simulink model "A3_control_loop_lin_d_model"  (Simulink 8.7)
settings: Solver=VariableStepDiscrete  StartTime=0.0  StopTime=5  MaxStep=1e-3  RelTol=1e-3
values from neighbouring files (symbols this model uses):
  H = sum_H * lin_sys.b    [a2_main.m]    (also in a3_main.m; a4_main.m)
  K_I = 0.31    [a3_main.m]    (also in a4_main.m)
  K_M = 1/63000    (= 1.5873015873e-05)    [a1_main.m]    (also in a2_main.m; a3_main.m; a4_main.m)
  lin_sys = linmod('A1_Hydropulszylinder',zeros(3,1),0)    [a1_main.m]    (also in a2_main.m; a3_main.m; a4_main.m)
  PHI = expm(Ta*lin_sys.a)    [a2_main.m]    (also in a3_main.m; a4_main.m)
  Ta = 15e-3    (= 0.015)    [a1_main.m]    (also in a2_main.m; a3_main.m; a4_main.m)
undefined symbols (not defined in the file or in its folder): DiscIntNeverNeededParam
libraries: simulink x1
settings Model: Creator=jinyao  LastModifiedBy=jinyao
settings DataIOCC: LimitDataPoints=off  SaveFormat=Dataset
settings DebuggingCC: UnderspecifiedInitializationDetection=Simplified  MergeDetectMultiDrivingBlocksExec=error
settings HardwareCC: ProdBitPerPointer=64  ProdLargestAtomicFloat=Float  ProdIntDivRoundTo=Zero  ProdEndianess=LittleEndian  ProdWordSize=64  ProdHWDeviceType=Intel->x86-64 (Windows64)
settings ModelReferenceCC: PropagateSignalLabelsOutOfModel=on
settings ConfigComp: CovModelRefEnable=off

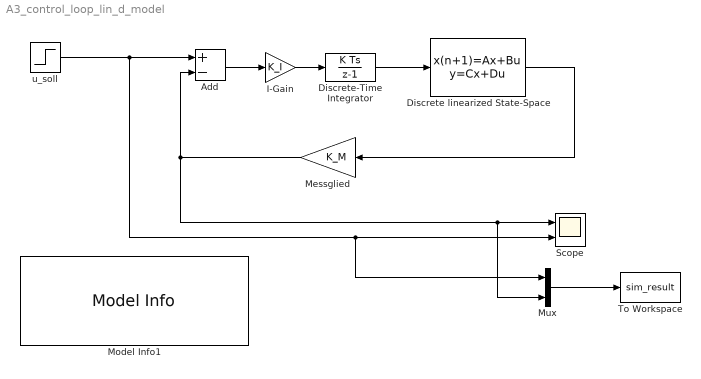
== system A3_control_loop_lin_d_model ==
  Add : Sum  Inputs=+-
  Discrete linearized State-Space : DiscreteStateSpace  A=PHI  B=H  C=lin_sys.c  D=0  SampleTime=Ta
  Discrete-Time Integrator : DiscreteIntegrator  InitialConditionSetting=State (most efficient)  SampleTime=Ta  ICPrevOutput=DiscIntNeverNeededParam  ICPrevScaledInput=DiscIntNeverNeededParam
  I-Gain : Gain  Gain=K_I
  Messglied : Gain  Gain=K_M
  Model Info1 : simulink/Model-Wide Utilities/Model Info  Frame=on  DisplayStringWithTags=|  HorizontalTextAlignment=Center  LeftAlignmentValue=0.5  SourceBlockDiagram=A3_control_loop_lin_d_model  TagMaxNumber=20
      | %<ModelName>
      | 
      | MODSIM GRUPPE 11
      | 
      | Cao,Bozhi  Gao,Yue  Jia,Xuehua  Zhu,Jinyao
      | 
      | 14.06.2018
  Mux : Mux  Inputs=2
  Scope : Scope  NumInputPorts=2
  To Workspace : ToWorkspace  VariableName=sim_result  SaveFormat=Structure With Time  SampleTime=-1
  u_soll : Step  After=0.5  SampleTime=0
  wires:
  Discrete-Time Integrator/1 -> Discrete linearized State-Space/1
  Discrete linearized State-Space/1 -> Messglied/1
  Messglied/1 -> Mux/2, Scope/1, Add/2
  Add/1 -> I-Gain/1
  u_soll/1 -> Mux/1, Scope/2, Add/1
  I-Gain/1 -> Discrete-Time Integrator/1
  Mux/1 -> To Workspace/1
